simulink model "Copy_of_sm_car_test_ggv_new"  (R2026a)
settings: Solver=ode23t  StopTime=300  MaxStep=0.4  AbsTol=1e-3  EnableMultiTasking=on
PreLoadFcn:
  | % PreLoadFcn Removed for GGV Sweep
PostLoadFcn:
  | % PostLoadFcn Removed for GGV Sweep
InitFcn:
  | sm_car_config_camera;
  | Vehicle = sm_car_vehcfg_checkConfig(Vehicle);
  | sm_car_check_tire_model(bdroot);
StartFcn:
  | tic;
StopFcn:
  | Elapsed_Sim_Time = toc;
  | % disp(['Elapsed Sim Time = ' num2str(Elapsed_Sim_Time)]);
undefined symbols (not defined in the file): acc_theta, accel_ramp_rate, Axle1D, AxleIn, Camera, Control, drag_frc, Driver, Init, lift_frc, Maneuver, Pedal, Scene, ShaftL1, ShaftL2, ShaftR1, ShaftR2, Visual, X, xy_data_car_side, Y, Z
libraries: sm_lib x272, fl_lib x171, nesl_utility x139, simulink x58, simulink_extras x14, sdl_lib x14, SimscapeFluids_lib x7, dspsigops x4, Damper_Element x4, Tire_1x2x x4, ee_lib x3, Scene_Utilities x3
(part 6 of 21)

== system Copy_of_sm_car_test_ggv_new/Controller/TrqVec_FLC/Susp ==
  aSteerWheel : Inport
  vx : Inport  Port=2
  1-D Lookup Table : Lookup_n-D  NumberOfTableDimensions=1  BreakpointsForDimension1=Steer.Gain.vVehicle.Value  Table=Steer.Gain.n.Value  InterpMethod=Linear Lagrange  InternalRulePriority=Speed  RndMeth=Simplest
  Bus Creator{1..4} (4 alike) : BusCreator  Inputs=1
  Gain : Gain  Gain=3.6
  Product : Product
  Saturation : Saturate  UpperLimit=Steer.Limits.aUpper.Value  LowerLimit=Steer.Limits.aLower.Value  LinearizeAsGain=off  ZeroCross=off
  Transfer Fcn (with initial states) : simulink_extras/Additional Linear/Transfer Fcn (with initial states)  N=[1]  D="[1/Steer.fActuatorCutoff.Value  1]"  X0=-1
  SuspA1 : Outport  VectorParamsAs1DForOutWhenUnconnected=off
  SuspA2 : Outport  Port=2  VectorParamsAs1DForOutWhenUnconnected=off
  wires:
  Bus Creator4/1 -> Bus Creator1/1  "Steer"
  Bus Creator2/1 -> Bus Creator3/1  "Steer"
  Bus Creator3/1 -> SuspA2/1  "SuspA2"
  Bus Creator1/1 -> SuspA1/1  "SuspA1"
  aSteerWheel/1 -> Product/1, Bus Creator4/1  "aSteerWheel"
  Saturation/1 -> Bus Creator2/1  "aSteerWheel"
  vx/1 -> Gain/1
  Transfer Fcn (with initial states)/1 -> Product/2
  Product/1 -> Saturation/1
  Gain/1 -> 1-D Lookup Table/1
  1-D Lookup Table/1 -> Transfer Fcn (with initial states)/1

== system Copy_of_sm_car_test_ggv_new/Controller/TrqVec_FLC_V2/Brake Control ==
  "rBrakePedal " : Inport
  "VehBus " : Inport  Port=2
  Pedal : Subsystem  VariantControl=Pedal
  " Brakes" : Outport  VectorParamsAs1DForOutWhenUnconnected=off

== system Copy_of_sm_car_test_ggv_new/Controller/TrqVec_FLC_V2/Driveline Control ==
  Bus Creator : BusCreator  Inputs=1
  Constant : Constant  Value=0
  Driveline : Outport  VectorParamsAs1DForOutWhenUnconnected=off
  wires:
  Constant/1 -> Bus Creator/1  "placeholder"
  Bus Creator/1 -> Driveline/1  "Driveline"

== system Copy_of_sm_car_test_ggv_new/Controller/TrqVec_FLC_V2/Power Control ==
  rAccelPedal : Inport
  VehBus : Inport  Port=2
  aSteerWheel : Inport  Port=3
  Bus Creator : BusCreator  Inputs=2
  Bus Selector : BusSelector  OutputSignals=Chassis.Body.CG.vx,Chassis.Body.CG.gx,Chassis.Body.CG.gy,Chassis.Body.CG.nYaw,Chassis.SuspA2.LinkageL.Upright.Upright.w,Chassis.SuspA2.LinkageR.Upright.Upright.w,Chassis.Body.CG.vy
  Controler type : Constant  Value=2
  Gain : Gain  Gain=max(Control.MotorTrq)
  Gain1 : Gain  Gain=max(Control.MotorTrq)
  Gain2 : Gain  Gain=1/9.80665
  TV FLC V2 : Subsystem  TreatAsAtomicUnit=on  ReferencedSubsystem=TV_FLC_V2  MotorT=Control.MotorTrq  Gr=Control.GearRatio  MotorW=Control.MotorW  rwheel=Control.WheelRad  tr=Control.RearTrack  a=Control.FrontTrackToCG  a_cop=Control.FrontTrackToCoP  Af=Control.FrontalArea  cd=Control.LiftCoef  g=Control.GravitationalAcc  ro=Control.AirDensity  m=Control.Mass  h_CG=Control.CGHeight  L=Control.Wheelbase  Gain=Control.StrWheelRatio  Ku=Control.UndersteerGradient  F=Control.F  P=Control.Proportional_P  I=Control.Integral_I  D=Control.Derivative_D  N=Control.Filter_N  Load_Ref=Control.LoadRef  Slip_Ref=Control.SlipRef  FIS_1=Control.FuzzySystem_1  FIS_2=Control.FuzzySystem_2  FIS_3=Control.FuzzySystem_3  vx_th=Control.ActivationVelocity  Tmax=max(Control.MotorTrq)  C_alpha_F=Control.CalphaF
  Power : Outport  VectorParamsAs1DForOutWhenUnconnected=off
  wires:
  aSteerWheel/1 -> TV FLC V2/1
  Gain2/1 -> TV FLC V2/4
  Gain1/1 -> Bus Creator/2  "MMotorR2Demand"
  Gain/1 -> Bus Creator/1  "MMotorL2Demand"
  TV FLC V2/2 -> Gain1/1  "MMotorR2Demand"
  TV FLC V2/1 -> Gain/1  "MMotorL2Demand"
  Bus Creator/1 -> Power/1
  rAccelPedal/1 -> TV FLC V2/9  "Throttle[~]"
  Bus Selector/6 -> TV FLC V2/7  "<w>"
  Bus Selector/5 -> TV FLC V2/6  "<w>"
  Bus Selector/4 -> TV FLC V2/5  "<nYaw>"
  Bus Selector/3 -> Gain2/1  "<gy>"
  Bus Selector/1 -> TV FLC V2/2  "<vx>"
  VehBus/1 -> Bus Selector/1
  Bus Selector/2 -> TV FLC V2/3  "<gx>"
  Bus Selector/7 -> TV FLC V2/8  "<vy>"
  Controler type/1 -> TV FLC V2/10

== system Copy_of_sm_car_test_ggv_new/Controller/TrqVec_FLC_V2/Spring Damper ==
  Bus Creator : BusCreator  Inputs=4
  Bus Creator1 : BusCreator  Inputs=4
  Constant : Constant  Value=[0 0 0 0]
  Constant1 : Constant  Value=[0 0 0 0]
  Demux : Demux
  Demux1 : Demux
  Damper : Outport  VectorParamsAs1DForOutWhenUnconnected=off
  Spring : Outport  Port=2  VectorParamsAs1DForOutWhenUnconnected=off
  wires:
  Bus Creator/1 -> Spring/1  "Spring"
  Bus Creator1/1 -> Damper/1  "Damper"
  Constant1/1 -> Demux1/1
  Demux1/3 -> Bus Creator1/3  "L2"
  Demux1/4 -> Bus Creator1/4  "R2"
  Demux1/1 -> Bus Creator1/1  "L1"
  Demux1/2 -> Bus Creator1/2  "R1"
  Demux/2 -> Bus Creator/2  "R1"
  Demux/1 -> Bus Creator/1  "L1"
  Demux/4 -> Bus Creator/4  "R2"
  Demux/3 -> Bus Creator/3  "L2"
  Constant/1 -> Demux/1

== system Copy_of_sm_car_test_ggv_new/Controller/TrqVec_FLC_V2/Susp ==
  aSteerWheel : Inport
  vx : Inport  Port=2
  1-D Lookup Table : Lookup_n-D  NumberOfTableDimensions=1  BreakpointsForDimension1=Steer.Gain.vVehicle.Value  Table=Steer.Gain.n.Value  InterpMethod=Linear Lagrange  InternalRulePriority=Speed  RndMeth=Simplest
  Bus Creator{1..4} (4 alike) : BusCreator  Inputs=1
  Gain : Gain  Gain=3.6
  Product : Product
  Saturation : Saturate  UpperLimit=Steer.Limits.aUpper.Value  LowerLimit=Steer.Limits.aLower.Value  LinearizeAsGain=off  ZeroCross=off
  Transfer Fcn (with initial states) : simulink_extras/Additional Linear/Transfer Fcn (with initial states)  N=[1]  D="[1/Steer.fActuatorCutoff.Value  1]"  X0=-1
  SuspA1 : Outport  VectorParamsAs1DForOutWhenUnconnected=off
  SuspA2 : Outport  Port=2  VectorParamsAs1DForOutWhenUnconnected=off
  wires:
  1-D Lookup Table/1 -> Transfer Fcn (with initial states)/1
  Gain/1 -> 1-D Lookup Table/1
  Product/1 -> Saturation/1
  Transfer Fcn (with initial states)/1 -> Product/2
  vx/1 -> Gain/1
  Saturation/1 -> Bus Creator2/1  "aSteerWheel"
  aSteerWheel/1 -> Bus Creator4/1, Product/1  "aSteerWheel"
  Bus Creator1/1 -> SuspA1/1  "SuspA1"
  Bus Creator3/1 -> SuspA2/1  "SuspA2"
  Bus Creator2/1 -> Bus Creator3/1  "Steer"
  Bus Creator4/1 -> Bus Creator1/1  "Steer"

== system Copy_of_sm_car_test_ggv_new/Controller/TrqVec_FLC_V3/Brake Control ==
  "rBrakePedal " : Inport
  "VehBus " : Inport  Port=2
  Pedal : Subsystem  VariantControl=Pedal
  " Brakes" : Outport  VectorParamsAs1DForOutWhenUnconnected=off

== system Copy_of_sm_car_test_ggv_new/Controller/TrqVec_FLC_V3/Driveline Control ==
  Bus Creator : BusCreator  Inputs=1
  Constant : Constant  Value=0
  Driveline : Outport  VectorParamsAs1DForOutWhenUnconnected=off
  wires:
  Bus Creator/1 -> Driveline/1  "Driveline"
  Constant/1 -> Bus Creator/1  "placeholder"

== system Copy_of_sm_car_test_ggv_new/Controller/TrqVec_FLC_V3/Power Control ==
  rAccelPedal : Inport
  VehBus : Inport  Port=2
  aSteerWheel : Inport  Port=3
  Bus Creator : BusCreator  Inputs=2
  Bus Selector : BusSelector  OutputSignals=Chassis.SuspA2.LinkageL.Upright.Upright.w,Chassis.SuspA2.LinkageR.Upright.Upright.w
  Bus Selector1 : BusSelector  OutputSignals=v_x,a_x,a_y,phi_dot,v_y
  Data Type Conversion{,1..8} (9 alike) : DataTypeConversion  OutDataTypeStr=single  SaturateOnIntegerOverflow=off  RndMeth=Floor
  Data Type Conversion10 : DataTypeConversion  OutDataTypeStr=double  SaturateOnIntegerOverflow=off  RndMeth=Floor
  Data Type Conversion11 : DataTypeConversion  OutDataTypeStr=double  SaturateOnIntegerOverflow=off  RndMeth=Floor
  Gain : Gain  Gain=max(Control.MotorTrq)
  Gain1 : Gain  Gain=max(Control.MotorTrq)
  TV FLC V3 : Subsystem  TreatAsAtomicUnit=on  ReferencedSubsystem=TV_FLC_V3  MotorT=Control.MotorTrq  Gr=Control.GearRatio  MotorW=Control.MotorW  rwheel=Control.WheelRad  tr=Control.RearTrack  a=Control.FrontTrackToCG  a_cop=Control.FrontTrackToCoP  Af=Control.FrontalArea  cd=Control.LiftCoef  Value=Control.GravitationalAcc  ro=Control.AirDensity  m=Control.Mass  h_CG=Control.CGHeight  L=Control.Wheelbase  StrWhlR=Control.StrWheelRatio  Ku=Control.UndersteerGradient  F=Control.F  Slip_Ctrl_Kp=70  Slip_Ctrl_Ki=150  Slip_Ctrl_Kd=1.5  Slip_Ctrl_Kn=Control.Filter_N  Load_Ref=Control.LoadRef  Slip_Ref=Control.SlipRef  FIS=Control.FuzzySystem  vx_th=Control.ActivationVelocity  Tmax=max(Control.MotorTrq)  C_alpha_F=Control.CalphaF  Slip_Steer_th=10  Kp_TV_Yaw=Control.Kp_Yaw  Kp_TV_Beta=Control.Kp_beta
  UKF State Estimation : Subsystem
  Power : Outport  VectorParamsAs1DForOutWhenUnconnected=off
  Out Bus Element : Outport  Port=2  PortName=Meas  Element=DYC
  Out Bus Element1 : Outport  Port=2  PortName=Meas  Element=UKF
  wires:
  VehBus/1 -> Bus Selector/1, UKF State Estimation/2(VehBus)
  Bus Selector/1 -> Data Type Conversion5/1  "<w>"
  Bus Selector/2 -> Data Type Conversion6/1  "<w>"
  rAccelPedal/1 -> Data Type Conversion8/1  "Throttle[~]"
  Bus Creator/1 -> Power/1
  TV FLC V3/1 -> Data Type Conversion10/1
  Gain/1 -> Bus Creator/1  "MMotorL2Demand"
  Gain1/1 -> Bus Creator/2  "MMotorR2Demand"
  aSteerWheel/1 -> Data Type Conversion/1, UKF State Estimation/1(aSteerWheel)
  TV FLC V3/2 -> Data Type Conversion11/1
  Data Type Conversion/1 -> TV FLC V3/1
  Data Type Conversion1/1 -> TV FLC V3/2
  Data Type Conversion2/1 -> TV FLC V3/3
  Data Type Conversion3/1 -> TV FLC V3/4
  Data Type Conversion4/1 -> TV FLC V3/5
  Data Type Conversion5/1 -> TV FLC V3/7
  Data Type Conversion6/1 -> TV FLC V3/8
  Data Type Conversion7/1 -> TV FLC V3/6
  Data Type Conversion8/1 -> TV FLC V3/9
  Data Type Conversion10/1 -> Gain/1
  Data Type Conversion11/1 -> Gain1/1
  TV FLC V3/3 -> Out Bus Element/1
  UKF State Estimation/1(StateEst) -> Bus Selector1/1
  Bus Selector1/1 -> Data Type Conversion1/1  "<v_x>"
  Bus Selector1/4 -> Data Type Conversion4/1  "<phi_dot>"
  Bus Selector1/2 -> Data Type Conversion2/1  "<a_x>"
  Bus Selector1/3 -> Data Type Conversion3/1  "<a_y>"
  Bus Selector1/5 -> Data Type Conversion7/1  "<v_y>"
  UKF State Estimation/2(Meas) -> Out Bus Element1/1  "Estimation"

== system Copy_of_sm_car_test_ggv_new/Controller/TrqVec_FLC_V3/Spring Damper ==
  Bus Creator : BusCreator  Inputs=4
  Bus Creator1 : BusCreator  Inputs=4
  Constant : Constant  Value=[0 0 0 0]
  Constant1 : Constant  Value=[0 0 0 0]
  Demux : Demux
  Demux1 : Demux
  Damper : Outport  VectorParamsAs1DForOutWhenUnconnected=off
  Spring : Outport  Port=2  VectorParamsAs1DForOutWhenUnconnected=off
  wires:
  Constant/1 -> Demux/1
  Demux/3 -> Bus Creator/3  "L2"
  Demux/4 -> Bus Creator/4  "R2"
  Demux/1 -> Bus Creator/1  "L1"
  Demux/2 -> Bus Creator/2  "R1"
  Demux1/2 -> Bus Creator1/2  "R1"
  Demux1/1 -> Bus Creator1/1  "L1"
  Demux1/4 -> Bus Creator1/4  "R2"
  Demux1/3 -> Bus Creator1/3  "L2"
  Constant1/1 -> Demux1/1
  Bus Creator1/1 -> Damper/1  "Damper"
  Bus Creator/1 -> Spring/1  "Spring"

== system Copy_of_sm_car_test_ggv_new/Controller/TrqVec_FLC_V3/Susp ==
  aSteerWheel : Inport
  vx : Inport  Port=2
  1-D Lookup Table : Lookup_n-D  NumberOfTableDimensions=1  BreakpointsForDimension1=Steer.Gain.vVehicle.Value  Table=Steer.Gain.n.Value  InterpMethod=Linear Lagrange  InternalRulePriority=Speed  RndMeth=Simplest
  Bus Creator{1..4} (4 alike) : BusCreator  Inputs=1
  Gain : Gain  Gain=3.6
  Product : Product
  Saturation : Saturate  UpperLimit=Steer.Limits.aUpper.Value  LowerLimit=Steer.Limits.aLower.Value  LinearizeAsGain=off  ZeroCross=off
  Transfer Fcn (with initial states) : simulink_extras/Additional Linear/Transfer Fcn (with initial states)  N=[1]  D="[1/Steer.fActuatorCutoff.Value  1]"  X0=-1
  SuspA1 : Outport  VectorParamsAs1DForOutWhenUnconnected=off
  SuspA2 : Outport  Port=2  VectorParamsAs1DForOutWhenUnconnected=off
  wires:
  Bus Creator4/1 -> Bus Creator1/1  "Steer"
  Bus Creator2/1 -> Bus Creator3/1  "Steer"
  Bus Creator3/1 -> SuspA2/1  "SuspA2"
  Bus Creator1/1 -> SuspA1/1  "SuspA1"
  aSteerWheel/1 -> Product/1, Bus Creator4/1  "aSteerWheel"
  Saturation/1 -> Bus Creator2/1  "aSteerWheel"
  vx/1 -> Gain/1
  Transfer Fcn (with initial states)/1 -> Product/2
  Product/1 -> Saturation/1
  Gain/1 -> 1-D Lookup Table/1
  1-D Lookup Table/1 -> Transfer Fcn (with initial states)/1

== system Copy_of_sm_car_test_ggv_new/Driver/Closed Loop/Driver ==
  vx : Inport
  Ref : Inport  Port=2
  CurPose : Inport  Port=3
  Preview : Inport  Port=4
  Bus Creator5 : BusCreator  Inputs=4
  Bus Selector1 : BusSelector  OutputSignals=vTarget
  Constant : Constant  Value=0.8
  Constant1 : Constant  Value=0
  Constant9 : Constant  Value=0
  Cur Pose : Subsystem
  Filter Steer Cmd : TransferFcn  Denominator=[1/Driver.Lateral.fSteerCutoff.Value 1]
  Fwd Rev : Subsystem
  Gain : Gain  Gain=5.71
  Lateral Driver : Subsystem  Variant=on  VariantControlMode=label  VariantControl=Choice  LabelModeActiveChoice=Pure_Pursuit  mask{Lateral=Driver.Lateral, VariantLabel=Driver.Lateral.class.Value}
      mask prompts: Lateral "Lateral Driver Parameters (structure)"; VariantLabel "Variant Label"
      mask init:
      | curblk = gcb;
      | 
      | % Set variant for this block 
      | set_param(curblk,'LabelModeActiveChoice',VariantLabel);
  Longitudinal Driver1 : autolibshared/Longitudinal Driver  extAccelOvr=off  extDecelOvr=off  extAccelHld=off  extDecelHld=off  extAccelZero=off  extDecelZero=off  cntrlType=Predictive  shftType=None  velUnits=m/s  gearOut=off  Kp=15  Ki=1  Kff=.05  Kg=.01  VehVelVec=[0 100]  KffVec=[.1 .1]  KpVec=[10 10]  KiVec=[5 5]  KgVec=[0 0]  m=265  Kpt=Driver.Long.FTractive.Value  tau=Driver.Long.tDriver.Value  L=0.1  aR=Driver.Long.NDragRoll.Value  bR=Driver.Long.NDragAero.Value  cR=Driver.Long.NDragAero.Value  g=Driver.Long.gGravity.Value  vnom=100  Kaw=.1  tauerr=.03  tauPt=2  GearInit=0  tShift=.1  pdlVec=[0.1 0.4 0.5 0.9]  upShftTbl=[-1 12.9375 26.4375 39.9375 51.18749999999999 62.4375 72.84375 83.25;-1 16.3125 29.8125 43.3125 54.5624 65.8125 76.78125 87.75;-1 19.6875 33.1875 46.68749999999999 57.9375 69.1875 80.71875 92.25;-1 33 52.5 77.25 100.5 138.75 161.875 185]  dwnShftTbl=[1 9.5625 23.0625 36.5625 47.8125 59.0625 68.90625 78.75;1 12.9375 26.4375 39.9375 51.18749999999999 62.4375 72.84375 83.25;1 16.3125 29.8125 43.3125 54.562499 65.8125 76.78125 87.75;1 19.6875 33.1875 46.68749999999999 57.9375 69.1875 80.71875 92.25]  tClutch=.5  tRev=.5  tPark=120  aMode=1  UpGearVec="[0  1  2  3  4  5  6  7]"  DownGearVec="[1  2  3  4  5  6  7  8]"
  Ref Pose and Distance : Subsystem
  Step : Step  Time=6  InitialValue=0.2  FinalValue=0.8  SampleTime=0
  Terminator{,1,3..4} (4 alike) : Terminator
  Transfer Fcn : TransferFcn  Denominator=[1/(Driver.Long.fAccelCutoff.Value) 1]
  Transfer Fcn1 : TransferFcn  Denominator=[1/(Driver.Long.fBrakeCutoff.Value) 1]
  DrvBus : Outport  VectorParamsAs1DForOutWhenUnconnected=off
  wires:
  Fwd Rev/2(vxFwRv) -> Longitudinal Driver1/2
  Bus Selector1/1 -> Longitudinal Driver1/1, Fwd Rev/2(vT)  "<vTarget>"
  Ref Pose and Distance/2(Dist) -> Lateral Driver/2(Distance)
  Preview/1 -> Lateral Driver/5(Preview)
  Lateral Driver/1(steeringAngle) -> Gain/1
  Fwd Rev/1(dir) -> Lateral Driver/6(Direction)
  vx/1 -> Fwd Rev/1(vx), Lateral Driver/4(v_x)
  Cur Pose/1(CurPose) -> Lateral Driver/3(currentPose)
  CurPose/1 -> Cur Pose/1(Cur)
  Constant9/1 -> Longitudinal Driver1/3
  Bus Creator5/1 -> DrvBus/1  "DrvBus"
  Longitudinal Driver1/2 -> Transfer Fcn/1
  Longitudinal Driver1/3 -> Transfer Fcn1/1
  Transfer Fcn1/1 -> Bus Creator5/4  "rBrakePedal"
  Ref/1 -> Bus Creator5/1, Bus Selector1/1, Ref Pose and Distance/1(Ref)
  Ref Pose and Distance/1(RefPose) -> Lateral Driver/1(referencePose)
  Filter Steer Cmd/1 -> Bus Creator5/2  "aSteerWheel"
  Longitudinal Driver1/1 -> Terminator/1
  Gain/1 -> Filter Steer Cmd/1
  Constant1/1 -> Terminator3/1  "rBrakePedal"
  Step/1 -> Terminator4/1  "rAccelPedal"
  Transfer Fcn/1 -> Bus Creator5/3  "rAccelPedal"
  Constant/1 -> Terminator1/1  "rAccelPedal"

== system Copy_of_sm_car_test_ggv_new/Driver/Closed Loop/Driver Override ==
  In : Inport
  None : Subsystem  VariantControl=None
  Override : Subsystem  VariantControl=Override
  DrvBus : Outport

== system Copy_of_sm_car_test_ggv_new/Driver/Closed Loop/Maneuver ==
  note: Fwd or
      | Rev
  VehBus : Inport
  Override : Inport  Port=2
  Abs : Abs  ZeroCross=off  SaturateOnIntegerOverflow=off
  Bus Creator : BusCreator  Inputs=7
  Bus Creator1 : BusCreator  Inputs=5
  Bus Selector : BusSelector  OutputSignals=World.x,World.y,World.z,World.aRoll,World.aPitch,World.aYaw,Chassis.Body.CG.vx
  Bus Selector1 : BusSelector  OutputSignals=x,y,z,vx
  Bus Selector2 : BusSelector  OutputSignals=Chassis.Body.CG.vx
  Bus Selector3 : BusSelector  OutputSignals=y,x,nLap,ayaw
  Constant : Constant  Value=-1
  Constant6 : Constant  Value=Maneuver.Trajectory.xTrajectory.Value
  Constant8 : Constant  Value=Maneuver.Trajectory.aYaw.Value
  Count Lap : Subsystem
  MATLAB Function : MATLAB Function  SystemSampleTime=0.1  mask{nPreviewPoints=Maneuver.nPreviewPoints.Value}
      mask prompts: nPreviewPoints "Number of Preview Points"
  Max Lateral Distance (m) : Constant  Value=Maneuver.xMaxLat.Value
  Memory : Memory  InitialCondition=-1
  Min Target Speed (m/s) : Constant  Value=Maneuver.vMinTarget.Value
  Mux : Mux  Inputs=3
  Mux1 : Mux  Inputs=3
  PoseTarget Visual : Subsystem
  Switch : Switch  Criteria=u2 > Threshold  SaturateOnIntegerOverflow=off  InputSameDT=off
  Target Speed Gain : Constant  Value=Maneuver.vGain.Value
  Window of Points to Check : Constant  Value=10
  preview distance : Lookup_n-D  NumberOfTableDimensions=1  BreakpointsForDimension1=Maneuver.xPreview.v.Value  Table=Maneuver.xPreview.x.Value  InternalRulePriority=Speed  RndMeth=Simplest
  vx override : Subsystem
  window only : Constant  Value=0
  x override : Subsystem
  y override : Subsystem
  z override : Subsystem
  vx : Outport  VectorParamsAs1DForOutWhenUnconnected=off
  Ref : Outport  Port=2  VectorParamsAs1DForOutWhenUnconnected=off
  CurPose : Outport  Port=3  VectorParamsAs1DForOutWhenUnconnected=off
  Preview : Outport  Port=4  VectorParamsAs1DForOutWhenUnconnected=off
  simres : Outport  Port=5  VectorParamsAs1DForOutWhenUnconnected=off
  wires:
  MATLAB Function/14(pp_preview_speed_pts) -> Bus Creator1/5  "pp_preview_speed_pts"
  MATLAB Function/1(ref_z) -> PoseTarget Visual/1(ref_z)
  Bus Selector3/4 -> PoseTarget Visual/5(ref_ayaw)  "<ayaw>"
  Bus Selector3/3 -> PoseTarget Visual/4(Lap Count)  "<nLap>"
  Bus Selector3/2 -> PoseTarget Visual/3(ref_x)  "<x>"
  Bus Selector3/1 -> PoseTarget Visual/2(ref_y)  "<y>"
  Count Lap/1(lapC) -> Bus Creator/1  "nLap"
  Bus Selector2/1 -> vx/1  "<vx>"
  VehBus/1 -> Bus Selector/1, Bus Selector2/1
  Bus Creator1/1 -> Preview/1  "lookahead"
  MATLAB Function/13(pp_preview_dist_pts) -> Bus Creator1/4  "pp_preview_dist_pts"
  MATLAB Function/12(pp_preview_yaw_pts) -> Bus Creator1/3  "pp_preview_yaw_pts"
  MATLAB Function/11(pp_preview_y_pts) -> Bus Creator1/2  "pp_preview_y_pts"
  MATLAB Function/10(pp_preview_x_pts) -> Bus Creator1/1  "pp_preview_x_pts"
  MATLAB Function/7(ld) -> Bus Creator/7  "latdev"
  Min Target Speed (m/s)/1 -> MATLAB Function/12(minSpd)
  Target Speed Gain/1 -> MATLAB Function/13(speedGain)
  Max Lateral Distance (m)/1 -> MATLAB Function/11(maxld)
  Bus Selector/1 -> Mux/1  "<x>"
  Bus Selector/6 -> Mux1/3  "<aYaw>"
  Bus Selector/4 -> Mux1/1  "<aRoll>"
  Constant8/1 -> MATLAB Function/8(yaw)
  Bus Selector/7 -> Abs/1  "<vx>"
  Mux1/1 -> MATLAB Function/2(q)
  Bus Selector/5 -> Mux1/2  "<aPitch>"
  Constant6/1 -> MATLAB Function/9(dist)
  Mux/1 -> MATLAB Function/1(p)
  Bus Selector/3 -> Mux/3  "<z>"
  y override/1(y_ovr) -> MATLAB Function/4(posy)
  Bus Selector/2 -> Mux/2  "<y>"
  MATLAB Function/3(ref_x) -> Bus Creator/3  "x"
  x override/1(x_ovr) -> MATLAB Function/3(posx)
  MATLAB Function/8(cp) -> CurPose/1  "CurPose"
  preview distance/1 -> MATLAB Function/10(pd)
  MATLAB Function/4(ref_y) -> Bus Creator/4  "y"
  MATLAB Function/5(ref_ayaw) -> Bus Creator/5  "ayaw"
  MATLAB Function/2(ad) -> Count Lap/1(ad), Bus Creator/2  "dist"
  Bus Creator/1 -> Bus Selector3/1, Ref/1  "Reference"
  MATLAB Function/6(vTarget) -> Bus Creator/6  "vTarget"
  MATLAB Function/9(simres) -> simres/1
  Window of Points to Check/1 -> MATLAB Function/7(xywin)
  MATLAB Function/15(idx_ptMin) -> Memory/1
  Switch/1 -> MATLAB Function/14(idx_ptMin_prev)
  Constant/1 -> Switch/3
  window only/1 -> Switch/2
  Memory/1 -> Switch/1
  z override/1(z_ovr) -> MATLAB Function/5(posz)
  Override/1 -> Bus Selector1/1
  Bus Selector1/4 -> vx override/1(vx)  "<vx>"
  vx override/1(vx_ovr) -> MATLAB Function/6(speed)
  Bus Selector1/3 -> z override/1(z)  "<z>"
  Bus Selector1/2 -> y override/1(y)  "<y>"
  Bus Selector1/1 -> x override/1(x)  "<x>"
  Abs/1 -> preview distance/1

== system Copy_of_sm_car_test_ggv_new/Driver/Closed Loop/Override ==
  "dist " : Inport
  "Obs " : Inport  Port=2
  None : Subsystem  VariantControl=None  mask(No Driver Override){override=Scene.Mallory_Park_Obstacle.Override}
      mask prompts: override "Override parameters (structure)"
      mask help: Driver commands are not overridden, regardless of inputs to subsystem.
  " Ovr" : Outport  VectorParamsAs1DForOutWhenUnconnected=off

== system Copy_of_sm_car_test_ggv_new/Driver/Closed Loop/Scopes ==
  <vx> : Inport
  Ref : Inport  Port=2
  CurPose : Inport  Port=3
  DrvBus : Inport  Port=4
  Bus Selector : BusSelector  OutputSignals=vTarget
  Bus Selector1 : BusSelector  OutputSignals=aSteerWheel,rAccelPedal,rBrakePedal
  Compare vx to Target : Scope  NumInputPorts=2
      settings: ActiveDisplayYMinimum=-4.79181  ActiveDisplayYMaximum=0.54534
  RefPose : Scope
      settings: ActiveDisplayYMinimum=-33.853108167875448  ActiveDisplayYMaximum=54.67797351087907
  Scope1 : Scope  NumInputPorts=3
      settings: ActiveDisplayYMinimum=-1.19495  ActiveDisplayYMaximum=0.13277  DataLoggingVariableName=ScopeData2
  wires:
  DrvBus/1 -> Bus Selector1/1
  Bus Selector1/1 -> Scope1/1  "<aSteerWheel>"
  Bus Selector1/2 -> Scope1/2  "<rAccelPedal>"
  <vx>/1 -> Compare vx to Target/1
  Bus Selector1/3 -> Scope1/3  "<rBrakePedal>"
  CurPose/1 -> RefPose/1
  Bus Selector/1 -> Compare vx to Target/2  "<vTarget>"
  Ref/1 -> Bus Selector/1

== system Copy_of_sm_car_test_ggv_new/Driver/Open Loop/Open Loop ==
  Bus Creator : BusCreator  Inputs=7
  Bus Creator5 : BusCreator  Inputs=4
  Constant : Constant  Value=10000
  Constant{1..6} (6 alike) : Constant  Value=0
  Input Sequence Accel Pedal : simulink/Sources/Repeating Sequence  rep_seq_t=Maneuver.Accel.t.Value  rep_seq_y=Maneuver.Accel.rPedal.Value
  Input Sequence Brake Pedal : simulink/Sources/Repeating Sequence  rep_seq_t=Maneuver.Brake.t.Value  rep_seq_y=Maneuver.Brake.rPedal.Value
  "Input Sequence Steering Wheel " : simulink/Sources/Repeating Sequence  rep_seq_t=Maneuver.Steer.t.Value  rep_seq_y=Maneuver.Steer.aWheel.Value
  DrvBus : Outport  VectorParamsAs1DForOutWhenUnconnected=off
  wires:
  Constant6/1 -> Bus Creator/7  "nLap"
  Constant/1 -> Bus Creator/1  "dist"
  Bus Creator/1 -> Bus Creator5/1  "Reference"
  Constant4/1 -> Bus Creator/5  "vTarget"
  Constant3/1 -> Bus Creator/4  "ayaw"
  Constant2/1 -> Bus Creator/3  "y"
  Constant5/1 -> Bus Creator/6  "latdev"
  Constant1/1 -> Bus Creator/2  "x"
  Input Sequence Accel Pedal/1 -> Bus Creator5/3  "rAccelPedal"
  "Input Sequence Steering Wheel "/1 -> Bus Creator5/2  "aSteerWheel"
  Input Sequence Brake Pedal/1 -> Bus Creator5/4  "rBrakePedal"
  Bus Creator5/1 -> DrvBus/1  "DrvBus"

== system Copy_of_sm_car_test_ggv_new/Road/Mu Scaling by Position/Scaling factors FL ==
  muX : Inport
  muY : Inport  Port=2
  s_LKX : Constant  Value=LKX
  s_LKY : Constant  Value=LKY
  s_LKYC : Constant  Value=LKYC
  s_LKZC : Constant  Value=LKZC
  s_LTR : Constant  Value=LTR
  scaling_vector : Mux  Inputs=7
  scaling : Outport  VectorParamsAs1DForOutWhenUnconnected=off
  wires:
  muX/1 -> scaling_vector/1
  s_LKX/1 -> scaling_vector/2
  muY/1 -> scaling_vector/3
  s_LKY/1 -> scaling_vector/4
  s_LKYC/1 -> scaling_vector/5
  s_LTR/1 -> scaling_vector/6
  s_LKZC/1 -> scaling_vector/7
  scaling_vector/1 -> scaling/1

== system Copy_of_sm_car_test_ggv_new/Road/Mu Scaling by Position/Scaling factors FR ==
  muX : Inport
  muY : Inport  Port=2
  s_LKX : Constant  Value=LKX
  s_LKY : Constant  Value=LKY
  s_LKYC : Constant  Value=LKYC
  s_LKZC : Constant  Value=LKZC
  s_LTR : Constant  Value=LTR
  scaling_vector : Mux  Inputs=7
  scaling : Outport  VectorParamsAs1DForOutWhenUnconnected=off
  wires:
  muX/1 -> scaling_vector/1
  s_LKX/1 -> scaling_vector/2
  muY/1 -> scaling_vector/3
  s_LKY/1 -> scaling_vector/4
  s_LKYC/1 -> scaling_vector/5
  s_LTR/1 -> scaling_vector/6
  s_LKZC/1 -> scaling_vector/7
  scaling_vector/1 -> scaling/1

== system Copy_of_sm_car_test_ggv_new/Road/Mu Scaling by Position/Scaling factors RL ==
  muX : Inport
  muY : Inport  Port=2
  s_LKX : Constant  Value=LKX
  s_LKY : Constant  Value=LKY
  s_LKYC : Constant  Value=LKYC
  s_LKZC : Constant  Value=LKZC
  s_LTR : Constant  Value=LTR
  scaling_vector : Mux  Inputs=7
  scaling : Outport  VectorParamsAs1DForOutWhenUnconnected=off
  wires:
  muX/1 -> scaling_vector/1
  s_LKX/1 -> scaling_vector/2
  muY/1 -> scaling_vector/3
  s_LKY/1 -> scaling_vector/4
  s_LKYC/1 -> scaling_vector/5
  s_LTR/1 -> scaling_vector/6
  s_LKZC/1 -> scaling_vector/7
  scaling_vector/1 -> scaling/1

== system Copy_of_sm_car_test_ggv_new/Road/Mu Scaling by Position/Scaling factors RR ==
  muX : Inport
  muY : Inport  Port=2
  s_LKX : Constant  Value=LKX
  s_LKY : Constant  Value=LKY
  s_LKYC : Constant  Value=LKYC
  s_LKZC : Constant  Value=LKZC
  s_LTR : Constant  Value=LTR
  scaling_vector : Mux  Inputs=7
  scaling : Outport  VectorParamsAs1DForOutWhenUnconnected=off
  wires:
  muX/1 -> scaling_vector/1
  s_LKX/1 -> scaling_vector/2
  muY/1 -> scaling_vector/3
  s_LKY/1 -> scaling_vector/4
  s_LKYC/1 -> scaling_vector/5
  s_LTR/1 -> scaling_vector/6
  s_LKZC/1 -> scaling_vector/7
  scaling_vector/1 -> scaling/1

== system Copy_of_sm_car_test_ggv_new/Road/Road Surface Height/None ==
  Chassis : Inport
  Bus Creator : BusCreator  Inputs=4
  Bus Creator1 : BusCreator  Inputs=4
  Constant : Constant  Value=[0 0 0 0]
  Constant{1..4} (4 alike) : Constant  Value=[0 0 1]
  Demux2 : Demux
  Signal Specification1 : SignalSpecification  Unit=m
  Terminator : Terminator
  gz : Outport  VectorParamsAs1DForOutWhenUnconnected=off
  uvec : Outport  Port=2  VectorParamsAs1DForOutWhenUnconnected=off
  wires:
  Bus Creator/1 -> uvec/1  "uvec"
  Constant4/1 -> Bus Creator/4  "R2"
  Constant1/1 -> Bus Creator/1  "L1"
  Constant2/1 -> Bus Creator/2  "R1"
  Constant3/1 -> Bus Creator/3  "L2"
  Demux2/3 -> Bus Creator1/3  "L2"
  Demux2/4 -> Bus Creator1/4  "R2"
  Demux2/2 -> Bus Creator1/2  "R1"
  Bus Creator1/1 -> gz/1  "gz"
  Signal Specification1/1 -> Demux2/1
  Demux2/1 -> Bus Creator1/1  "L1"
  Constant/1 -> Signal Specification1/1
  Chassis/1 -> Terminator/1

== system Copy_of_sm_car_test_ggv_new/Scopes/Combined Tire Usage/FL_Fcomb ==
  <Fx> : Inport
  <Fy> : Inport  Port=2
  <Fz> : Inport  Port=3
  <rMuX> : Inport  Port=4
  <rMuY> : Inport  Port=5
  Abs : Abs  SaturateOnIntegerOverflow=off
  Add : Sum
  Add1 : Sum
  Divide : Product  Inputs=*/
  Gain : Gain  Gain=100
  Product : Product
  Product1 : Product
  Safe Division : Bias  Bias=0.01  SaturateOnIntegerOverflow=off
  Square{,1,3..4} (4 alike) : Math  Operator=square
  Square Root : Sqrt
  Square Root1 : Sqrt
  Fcomb% : Outport
  wires:
  Abs/1 -> Fcomb%/1
  Add/1 -> Square Root/1
  Square1/1 -> Add/2
  <Fx>/1 -> Square/1
  <Fz>/1 -> Safe Division/1
  <Fy>/1 -> Square1/1
  Gain/1 -> Abs/1
  Square/1 -> Add/1
  Square Root/1 -> Divide/1
  <rMuX>/1 -> Product/1
  Product1/1 -> Square4/1
  Product/1 -> Square3/1
  Square3/1 -> Add1/1
  Divide/1 -> Gain/1
  Square4/1 -> Add1/2
  Add1/1 -> Square Root1/1
  Square Root1/1 -> Divide/2
  <rMuY>/1 -> Product1/2
  Safe Division/1 -> Product1/1, Product/2

== system Copy_of_sm_car_test_ggv_new/Scopes/Combined Tire Usage/FR_Fcomb ==
  <Fx> : Inport
  <Fy> : Inport  Port=2
  <Fz> : Inport  Port=3
  <rMuX> : Inport  Port=4
  <rMuY> : Inport  Port=5
  Abs : Abs  SaturateOnIntegerOverflow=off
  Add : Sum
  Add1 : Sum
  Divide : Product  Inputs=*/
  Gain : Gain  Gain=100
  Product : Product
  Product1 : Product
  Safe Division : Bias  Bias=0.01  SaturateOnIntegerOverflow=off
  Square{,1,3..4} (4 alike) : Math  Operator=square
  Square Root : Sqrt
  Square Root1 : Sqrt
  Fcomb% : Outport
  wires:
  Safe Division/1 -> Product/2, Product1/1
  <rMuY>/1 -> Product1/2
  Square Root1/1 -> Divide/2
  Add1/1 -> Square Root1/1
  Square4/1 -> Add1/2
  Divide/1 -> Gain/1
  Square3/1 -> Add1/1
  Product/1 -> Square3/1
  Product1/1 -> Square4/1
  <rMuX>/1 -> Product/1
  Square Root/1 -> Divide/1
  Square/1 -> Add/1
  Gain/1 -> Abs/1
  <Fy>/1 -> Square1/1
  <Fz>/1 -> Safe Division/1
  <Fx>/1 -> Square/1
  Square1/1 -> Add/2
  Add/1 -> Square Root/1
  Abs/1 -> Fcomb%/1

== system Copy_of_sm_car_test_ggv_new/Scopes/Combined Tire Usage/RL_Fcomb ==
  <Fx> : Inport
  <Fy> : Inport  Port=2
  <Fz> : Inport  Port=3
  <rMuX> : Inport  Port=4
  <rMuY> : Inport  Port=5
  Abs : Abs  SaturateOnIntegerOverflow=off
  Add : Sum
  Add1 : Sum
  Divide : Product  Inputs=*/
  Gain : Gain  Gain=100
  Product : Product
  Product1 : Product
  Safe Division : Bias  Bias=0.01  SaturateOnIntegerOverflow=off
  Square{,1,3..4} (4 alike) : Math  Operator=square
  Square Root : Sqrt
  Square Root1 : Sqrt
  Fcomb% : Outport
  wires:
  Abs/1 -> Fcomb%/1
  Add/1 -> Square Root/1
  Square1/1 -> Add/2
  <Fx>/1 -> Square/1
  <Fz>/1 -> Safe Division/1
  <Fy>/1 -> Square1/1
  Gain/1 -> Abs/1
  Square/1 -> Add/1
  Square Root/1 -> Divide/1
  <rMuX>/1 -> Product/1
  Product1/1 -> Square4/1
  Product/1 -> Square3/1
  Square3/1 -> Add1/1
  Divide/1 -> Gain/1
  Square4/1 -> Add1/2
  Add1/1 -> Square Root1/1
  Square Root1/1 -> Divide/2
  <rMuY>/1 -> Product1/2
  Safe Division/1 -> Product1/1, Product/2

== system Copy_of_sm_car_test_ggv_new/Scopes/Combined Tire Usage/RR_Fcomb ==
  <Fx> : Inport
  <Fy> : Inport  Port=2
  <Fz> : Inport  Port=3
  <rMuX> : Inport  Port=4
  <rMuY> : Inport  Port=5
  Abs : Abs  SaturateOnIntegerOverflow=off
  Add : Sum
  Add1 : Sum
  Divide : Product  Inputs=*/
  Gain : Gain  Gain=100
  Product : Product
  Product1 : Product
  Safe Division : Bias  Bias=0.01  SaturateOnIntegerOverflow=off
  Square{,1,3..4} (4 alike) : Math  Operator=square
  Square Root : Sqrt
  Square Root1 : Sqrt
  Fcomb% : Outport
  wires:
  Safe Division/1 -> Product/2, Product1/1
  <rMuY>/1 -> Product1/2
  Square Root1/1 -> Divide/2
  Add1/1 -> Square Root1/1
  Square4/1 -> Add1/2
  Divide/1 -> Gain/1
  Square3/1 -> Add1/1
  Product/1 -> Square3/1
  Product1/1 -> Square4/1
  <rMuX>/1 -> Product/1
  Square Root/1 -> Divide/1
  Square/1 -> Add/1
  Gain/1 -> Abs/1
  <Fy>/1 -> Square1/1
  <Fz>/1 -> Safe Division/1
  <Fx>/1 -> Square/1
  Square1/1 -> Add/2
  Add/1 -> Square Root/1
  Abs/1 -> Fcomb%/1

== system Copy_of_sm_car_test_ggv_new/Scopes/Lateral Tire Usage/FL_Y ==
  <Fy> : Inport
  <rMuY> : Inport  Port=2
  <Fz> : Inport  Port=3
  Abs : Abs  SaturateOnIntegerOverflow=off
  Divide : Product  Inputs=*/
  Gain : Gain  Gain=100
  Product : Product
  Safe Division : Bias  Bias=0.01  SaturateOnIntegerOverflow=off
  Fy% : Outport
  wires:
  Abs/1 -> Fy%/1
  Divide/1 -> Gain/1
  Product/1 -> Divide/2
  <Fy>/1 -> Divide/1
  <Fz>/1 -> Safe Division/1
  <rMuY>/1 -> Product/1
  Gain/1 -> Abs/1
  Safe Division/1 -> Product/2

== system Copy_of_sm_car_test_ggv_new/Scopes/Lateral Tire Usage/FR_Y ==
  <Fy> : Inport
  <rMuY> : Inport  Port=2
  <Fz> : Inport  Port=3
  Abs : Abs  SaturateOnIntegerOverflow=off
  Divide : Product  Inputs=*/
  Gain : Gain  Gain=100
  Product : Product
  Safe Division : Bias  Bias=0.01  SaturateOnIntegerOverflow=off
  Fy% : Outport
  wires:
  Abs/1 -> Fy%/1
  Divide/1 -> Gain/1
  Product/1 -> Divide/2
  <Fy>/1 -> Divide/1
  <Fz>/1 -> Safe Division/1
  <rMuY>/1 -> Product/1
  Gain/1 -> Abs/1
  Safe Division/1 -> Product/2

== system Copy_of_sm_car_test_ggv_new/Scopes/Lateral Tire Usage/RL_Y ==
  <Fy> : Inport
  <rMuY> : Inport  Port=2
  <Fz> : Inport  Port=3
  Abs : Abs  SaturateOnIntegerOverflow=off
  Divide : Product  Inputs=*/
  Gain : Gain  Gain=100
  Product : Product
  Safe Division : Bias  Bias=0.01  SaturateOnIntegerOverflow=off
  Fy% : Outport
  wires:
  Safe Division/1 -> Product/2
  Gain/1 -> Abs/1
  <rMuY>/1 -> Product/1
  <Fz>/1 -> Safe Division/1
  <Fy>/1 -> Divide/1
  Product/1 -> Divide/2
  Divide/1 -> Gain/1
  Abs/1 -> Fy%/1

== system Copy_of_sm_car_test_ggv_new/Scopes/Lateral Tire Usage/RR_Y ==
  <Fy> : Inport
  <rMuY> : Inport  Port=2
  <Fz> : Inport  Port=3
  Abs : Abs  SaturateOnIntegerOverflow=off
  Divide : Product  Inputs=*/
  Gain : Gain  Gain=100
  Product : Product
  Safe Division : Bias  Bias=0.01  SaturateOnIntegerOverflow=off
  Fy% : Outport
  wires:
  Abs/1 -> Fy%/1
  Divide/1 -> Gain/1
  Product/1 -> Divide/2
  <Fy>/1 -> Divide/1
  <Fz>/1 -> Safe Division/1
  <rMuY>/1 -> Product/1
  Gain/1 -> Abs/1
  Safe Division/1 -> Product/2

== system Copy_of_sm_car_test_ggv_new/Scopes/Longitudinal Tire Usage/RL_X ==
  <Fx> : Inport
  <rMuX> : Inport  Port=2
  <Fz> : Inport  Port=3
  Abs : Abs  SaturateOnIntegerOverflow=off
  Add Constant : Bias  Bias=0.01  SaturateOnIntegerOverflow=off
  Divide : Product  Inputs=*/
  Gain : Gain  Gain=100
  Product : Product
  Fx% : Outport
  wires:
  Gain/1 -> Abs/1
  <rMuX>/1 -> Product/1
  <Fz>/1 -> Add Constant/1
  <Fx>/1 -> Divide/1
  Product/1 -> Divide/2
  Divide/1 -> Gain/1
  Abs/1 -> Fx%/1
  Add Constant/1 -> Product/2

== system Copy_of_sm_car_test_ggv_new/Scopes/Longitudinal Tire Usage/RR_X ==
  <Fx> : Inport
  <rMuX> : Inport  Port=2
  <Fz> : Inport  Port=3
  Abs : Abs  SaturateOnIntegerOverflow=off
  Add Constant : Bias  Bias=0.01  SaturateOnIntegerOverflow=off
  Divide : Product  Inputs=*/
  Gain : Gain  Gain=100
  Product : Product
  Fx% : Outport
  wires:
  Add Constant/1 -> Product/2
  Abs/1 -> Fx%/1
  Divide/1 -> Gain/1
  Product/1 -> Divide/2
  <Fx>/1 -> Divide/1
  <Fz>/1 -> Add Constant/1
  <rMuX>/1 -> Product/1
  Gain/1 -> Abs/1

== system Copy_of_sm_car_test_ggv_new/Scopes/Stability Factor/Understeer Gradient Calculation ==
  VehBus : Inport
  Enable : EnablePort
  Add1 : Sum  Inputs=-+
  Bus Selector1 : BusSelector  OutputSignals=Chassis.SuspA1.Steer.aWheel,Chassis.Body.CG.vx,Chassis.Body.CG.nYaw,Chassis.Body.CG.gy
  Divide4 : Product  Inputs=/*
  Gain : Gain  Gain=1.575
  Gain1 : Gain  Gain=1/5.71
  Gain6 : Gain  Gain=1/9.81
  Product8 : Product  Inputs=*/
  K : Outport
  wires:
  VehBus/1 -> Bus Selector1/1
  Bus Selector1/1 -> Gain1/1  "<aWheel>"
  Bus Selector1/3 -> Divide4/2  "<nYaw>"
  Divide4/1 -> Gain/1
  Product8/1 -> K/1  "K"
  Gain/1 -> Add1/2
  Bus Selector1/2 -> Divide4/1  "<vx>"
  Bus Selector1/4 -> Gain6/1  "<gy>"
  Gain1/1 -> Add1/1
  Gain6/1 -> Product8/2
  Add1/1 -> Product8/1

== system Copy_of_sm_car_test_ggv_new/Scopes/Yaw Reference/Subsystem ==
  v_x : Inport
  aSteerWheel : Inport  Port=2
  a_y : Inport  Port=3
  Enable : EnablePort
  Abs : Abs  SaturateOnIntegerOverflow=off
  Add : Sum
  Add Constant : Bias  Bias=1e-3  SaturateOnIntegerOverflow=off
  Divide : Product  Inputs=/*
  Divide1 : Product  Inputs=**/
  Gain : Gain  Gain=-0.00012434
  Gain1 : Gain  Gain=-1
  Power : Math  Operator=square
  Saturation Dynamic : sl_discontinuities/Saturation Dynamic  OutMin=[]  OutMax=[]  OutDataTypeStr=Inherit: Same as second input  OutDataType=fixdt(1, 16)  OutScaling=2^-10  DoSatur=off
  StrWheelRatio : Gain  Gain=1/5.71
  Wheelbase : Constant  Value=1.578
  y : Outport
  wires:
  Saturation Dynamic/1 -> y/1
  aSteerWheel/1 -> StrWheelRatio/1
  StrWheelRatio/1 -> Divide1/1  "aWheel_rad"
  Divide1/1 -> Saturation Dynamic/2  "YawDesired"
  v_x/1 -> Power/1, Divide1/2, Add Constant/1
  Power/1 -> Gain/1
  Gain1/1 -> Saturation Dynamic/3
  Gain/1 -> Add/1
  Divide/1 -> Abs/1
  Wheelbase/1 -> Add/2
  Add/1 -> Divide1/3
  Abs/1 -> Gain1/1, Saturation Dynamic/1  "YawMax"
  a_y/1 -> Divide/2
  Add Constant/1 -> Divide/1

== system Copy_of_sm_car_test_ggv_new/Vehicle/Trailer/None ==
  note: Ports deliberately not connected. They are necessary for unit tests, but not necessary here.
  "RdBus " : Inport
  "DrvBus " : Inport  Port=2
  "CtrlBus " : Inport  Port=3
  Ground : Ground
  Reference Frame : sm_lib/Frames and Transforms/Reference Frame
  Terminator : Terminator
  Terminator1 : Terminator
  Terminator2 : Terminator
  " C" : PMIOPort  Side=Left
  " W" : PMIOPort  Port=2  Side=Left
  " Hitch" : PMIOPort  Port=3  Side=Right
  " VehBus" : Outport  VectorParamsAs1DForOutWhenUnconnected=off
  wires:
  "RdBus "/1 -> Terminator/1
  "DrvBus "/1 -> Terminator1/1
  "CtrlBus "/1 -> Terminator2/1
  Ground/1 -> " VehBus"/1
  connections:
  " Hitch"/RConn1 -- Reference Frame/RConn1

== system Copy_of_sm_car_test_ggv_new/Vehicle/Vehicle/A1 to World ==
  Body World Joint : sm_lib/Joints/6-DOF Joint  JointMode=Normal  CompositeWrenchDir=FollowerOnBase  CompositeWrenchFrame=BaseFrame  SenseConstraintForce=off  SenseConstraintTorque=off  SenseTotalForce=off  SenseTotalTorque=off  PxPositionTargetSpecify=off  PxPositionTargetPriority=Low  PxPositionTargetValue=Init.sChassis.Value(1)  PxPositionTargetValueUnits=m  PxVelocityTargetSpecify=off  PxVelocityTargetPriority=Low  PxVelocityTargetValue=initial_vveh(1)  PxVelocityTargetValueUnits=m/s  PxEquilibriumPosition=0  PxEquilibriumPositionUnits=m  PxSpringStiffness=0  PxSpringStiffnessUnits=N/m  PxDampingCoefficient=0  PxDampingCoefficientUnits=N/(m/s)  PxLowerLimitSpecify=off  PxLowerLimitBound=-1  PxLowerLimitBoundUnits=m  PxLowerLimitStiffness=1e6  PxLowerLimitStiffnessUnits=N/m  PxLowerLimitDamping=1e3  PxLowerLimitDampingUnits=N/(m/s)  PxLowerLimitTransitionRegionWidth=1e-4  PxLowerLimitTransitionRegionWidthUnits=m  PxUpperLimitSpecify=off  PxUpperLimitBound=1  PxUpperLimitBoundUnits=m  PxUpperLimitStiffness=1e6  PxUpperLimitStiffnessUnits=N/m  PxUpperLimitDamping=1e3  PxUpperLimitDampingUnits=N/(m/s)  PxUpperLimitTransitionRegionWidth=1e-4  PxUpperLimitTransitionRegionWidthUnits=m  PxTorqueActuationMode=NoTorque  PxMotionActuationMode=ComputedMotion  PxSensePosition=off  PxSenseVelocity=off  PxSenseAcceleration=off  PxSenseTorqueForce=off  PxSenseLowerLimitTorqueForce=off  PxSenseUpperLimitTorqueForce=off  PyPositionTargetSpecify=off  PyPositionTargetPriority=Low  PyPositionTargetValue=Init.sChassis.Value(2)  PyPositionTargetValueUnits=m  PyVelocityTargetSpecify=off  PyVelocityTargetPriority=Low  PyVelocityTargetValue=initial_vveh(2)  PyVelocityTargetValueUnits=m/s  PyEquilibriumPosition=0  PyEquilibriumPositionUnits=m  PySpringStiffness=0  PySpringStiffnessUnits=N/m  PyDampingCoefficient=0  PyDampingCoefficientUnits=N/(m/s)  PyLowerLimitSpecify=off  PyLowerLimitBound=-1  PyLowerLimitBoundUnits=m  PyLowerLimitStiffness=1e6  PyLowerLimitStiffnessUnits=N/m  PyLowerLimitDamping=1e3  PyLowerLimitDampingUnits=N/(m/s)  PyLowerLimitTransitionRegionWidth=1e-4  PyLowerLimitTransitionRegionWidthUnits=m  PyUpperLimitSpecify=off  PyUpperLimitBound=1  PyUpperLimitBoundUnits=m  PyUpperLimitStiffness=1e6  PyUpperLimitStiffnessUnits=N/m  PyUpperLimitDamping=1e3  PyUpperLimitDampingUnits=N/(m/s)  PyUpperLimitTransitionRegionWidth=1e-4  PyUpperLimitTransitionRegionWidthUnits=m  PyTorqueActuationMode=NoTorque  PyMotionActuationMode=ComputedMotion  PySensePosition=off  PySenseVelocity=off  PySenseAcceleration=off  PySenseTorqueForce=off  PySenseLowerLimitTorqueForce=off  PySenseUpperLimitTorqueForce=off  PzPositionTargetSpecify=off  PzPositionTargetPriority=Low  PzPositionTargetValue=Init.sChassis.Value(3)  PzPositionTargetValueUnits=m  PzVelocityTargetSpecify=off  PzVelocityTargetPriority=Low  PzVelocityTargetValue=initial_vveh(3)  PzVelocityTargetValueUnits=m/s  PzEquilibriumPosition=0  PzEquilibriumPositionUnits=m  PzSpringStiffness=0  PzSpringStiffnessUnits=N/m  PzDampingCoefficient=0  PzDampingCoefficientUnits=N/(m/s)  PzLowerLimitSpecify=off  PzLowerLimitBound=-1  PzLowerLimitBoundUnits=m  PzLowerLimitStiffness=1e6  PzLowerLimitStiffnessUnits=N/m  PzLowerLimitDamping=1e3  PzLowerLimitDampingUnits=N/(m/s)  PzLowerLimitTransitionRegionWidth=1e-4  PzLowerLimitTransitionRegionWidthUnits=m  PzUpperLimitSpecify=off  PzUpperLimitBound=1  PzUpperLimitBoundUnits=m  PzUpperLimitStiffness=1e6  PzUpperLimitStiffnessUnits=N/m  PzUpperLimitDamping=1e3  PzUpperLimitDampingUnits=N/(m/s)  PzUpperLimitTransitionRegionWidth=1e-4  PzUpperLimitTransitionRegionWidthUnits=m  PzTorqueActuationMode=NoTorque  PzMotionActuationMode=ComputedMotion  PzSensePosition=on  PzSenseVelocity=off  PzSenseAcceleration=off  PzSenseTorqueForce=off  PzSenseLowerLimitTorqueForce=off  PzSenseUpperLimitTorqueForce=off  SphPositionTargetSpecify=off  SphPositionTargetPriority=Low  SphPositionTargetRotationMethod=RotationSequence  SphPositionTargetFollAlignAxisA=+X  SphPositionTargetBaseAlignAxisA=+Y  SphPositionTargetFollAlignAxisB=+Y  SphPositionTargetBaseAlignAxisB=+Z  SphPositionTargetRotationStandardAxis=+Z  SphPositionTargetRotationAngle=0.0  SphPositionTargetRotationAngleUnits=deg  SphPositionTargetRotationArbitraryAxis=[0 0 1]  SphPositionTargetRotationSequenceAxes=FollowerAxes  SphPositionTargetRotationSequence=ZYX  SphPositionTargetRotationSequenceAngles=initial_aveh  SphPositionTargetRotationSequenceAnglesUnits=rad  SphPositionTargetRotationMatrix=[1 0 0; 0 1 0; 0 0 1]  SphPositionTargetQuaternion=[1 0 0 0]  SphVelocityTargetSpecify=off  SphVelocityTargetPriority=High  SphVelocityTargetValue=[0 0 0]  SphVelocityTargetValueUnits=deg/s  SphVelocityTargetInFollowerFrame=on  SphEqPosRotationMethod=None  SphEqPosFollAlignAxisA=+X  SphEqPosBaseAlignAxisA=+Y  SphEqPosFollAlignAxisB=+Y  SphEqPosBaseAlignAxisB=+Z  SphEqPosRotationStandardAxis=+Z  SphEqPosRotationAngle=0.0  SphEqPosRotationAngleUnits=deg  SphEqPosRotationArbitraryAxis=[0 0 1]  SphEqPosRotationSequenceAxes=FollowerAxes  SphEqPosRotationSequence=XYX  SphEqPosRotationSequenceAngles=[0 0 0]  SphEqPosRotationSequenceAnglesUnits=deg  SphEqPosRotationMatrix=[1 0 0; 0 1 0; 0 0 1]  SphEqPosQuaternion=[1 0 0 0]  SphSpringStiffness=0  SphSpringStiffnessUnits=N*m/deg  SphDampingCoefficient=0  SphDampingCoefficientUnits=N*m/(deg/s)  SphLowerLimitSpecify=off  SphLowerLimitBound=15  SphLowerLimitBoundUnits=deg  SphLowerLimitStiffness=1e4  SphLowerLimitStiffnessUnits=N*m/deg  SphLowerLimitDamping=10  SphLowerLimitDampingUnits=N*m/(deg/s)  SphLowerLimitTransitionRegionWidth=0.1  SphLowerLimitTransitionRegionWidthUnits=deg  SphUpperLimitSpecify=off  SphUpperLimitBound=45  SphUpperLimitBoundUnits=deg  SphUpperLimitStiffness=1e4  SphUpperLimitStiffnessUnits=N*m/deg  SphUpperLimitDamping=10  SphUpperLimitDampingUnits=N*m/(deg/s)  SphUpperLimitTransitionRegionWidth=0.1  SphUpperLimitTransitionRegionWidthUnits=deg  SphTorqueActuationMode=NoTorque  SphActuateTorqueX=off  SphActuateTorqueY=off  SphActuateTorqueZ=off  SphActuateTorque=off  SphActuationFrame=BaseFrame  SphSensePosition=off  SphSenseVelocityX=off  SphSenseVelocityY=off  SphSenseVelocityZ=off  SphSenseVelocity=off  SphSenseAccelerationX=off  SphSenseAccelerationY=off  SphSenseAccelerationZ=off  SphSenseAcceleration=off  SphSenseLowerLimitTorqueMag=off  SphSenseUpperLimitTorqueMag=off  SphSensingFrame=BaseFrame
  PS-Simulink Converter2 : nesl_utility/PS-Simulink Converter  PhysicalDomain=network_engine_domain  SubClassName=ps_output  LeftPortType=input  RightPortType=output  PseudoPeriodic=off  Frequencies=[]  VectorFormat=1-D array  Unit=m  AffineConversion=off
  Transform Sensor : sm_lib/Frames and Transforms/Transform Sensor  MeasurementFrame=World  RotationSequence=XYX  SenseAngle=off  SenseAxis=off  SenseQ=off  SenseR=off  SenseRotationSequence=off  SenseOmegaX=off  SenseOmegaY=off  SenseOmegaZ=off  SenseOmega=off  SenseQDot=off  SenseRDot=off  SenseRotationSequenceDot=off  SenseAlphaX=off  SenseAlphaY=off  SenseAlphaZ=off  SenseAlpha=off  SenseQDDot=off  SenseRDDot=off  SenseX=off  SenseY=off  SenseZ=off  SenseXYZ=off  SenseRad=off  SenseAzim=off  SenseDist=off  SenseInc=off  SenseXDot=off  SenseYDot=off  SenseZDot=off  SenseXYZDot=off  SenseRadDot=off  SenseAzimDot=off  SenseDistDot=off  SenseIncDot=off  SenseXDDot=off  SenseYDDot=off  SenseZDDot=off  SenseXYZDDot=off  SenseRadDDot=off  SenseAzimDDot=off  SenseDistDDot=off  SenseIncDDot=off
  F : PMIOPort  Side=Left
  B : PMIOPort  Port=2  Side=Right
  Bus Element Out6 : Outport  VectorParamsAs1DForOutWhenUnconnected=off  PortName=World  Element=z
  wires:
  PS-Simulink Converter2/1 -> Bus Element Out6/1
  connections:
  Body World Joint/RConn2 -- PS-Simulink Converter2/LConn1
  Body World Joint/RConn1 -- F/RConn1 -- Transform Sensor/RConn1
  Body World Joint/LConn1 -- B/RConn1 -- Transform Sensor/LConn1
